simulink library "simp_vd_lib"  (R2022b)
settings: Solver=VariableStepAuto  StartTime=0.0  StopTime=10.0  RelTol=1e-3
libraries: simulink x1
settings Model: Creator=LinF  LastModifiedBy=LinF

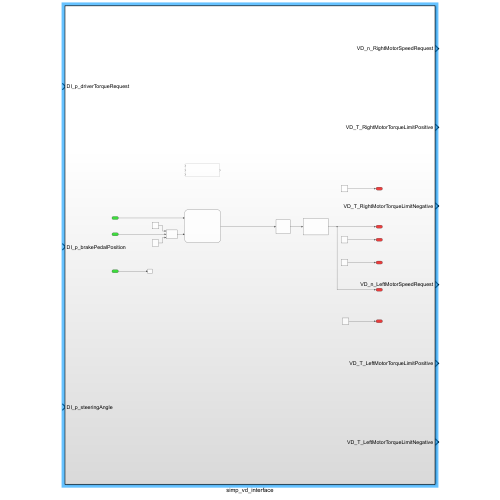
[thumbnail: Simulink's stored preview of the top-level diagram]
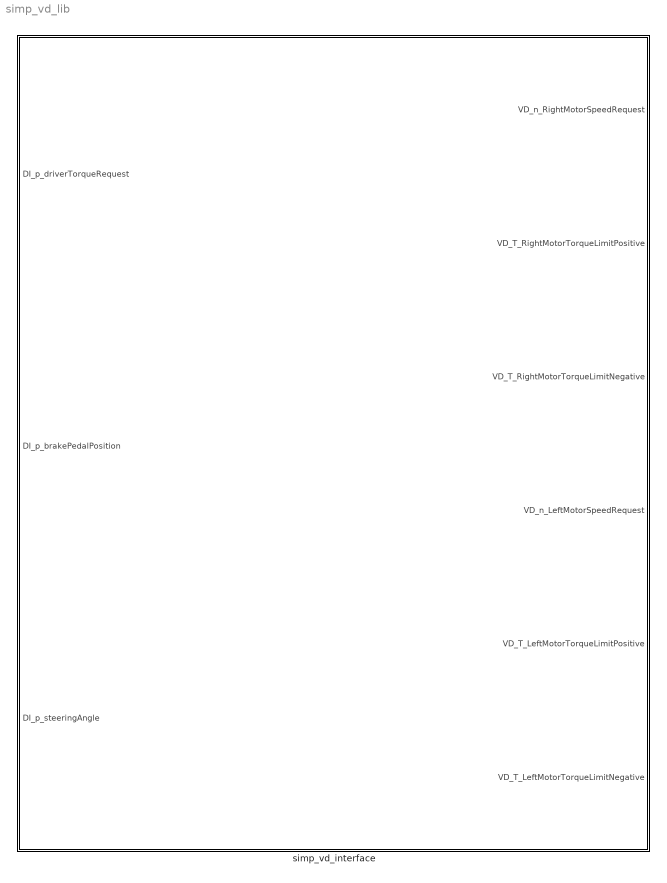
== system simp_vd_lib ==
  simp_vd_interface : Subsystem
      settings: LibrarySourceBlock=simp_vd_lib/simp_vd_interface

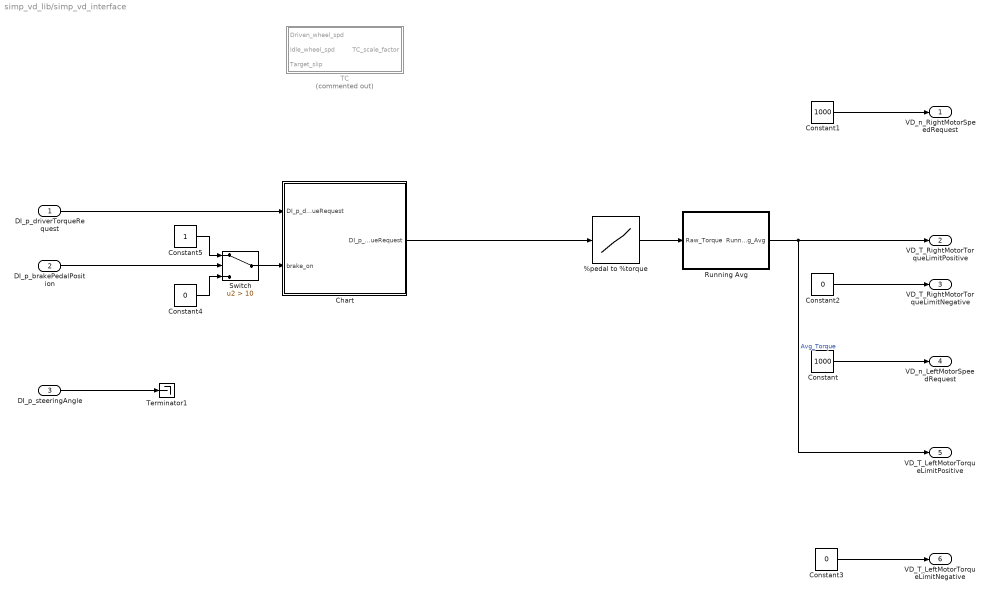
== system simp_vd_lib/simp_vd_interface ==
  DI_p_driverTorqueRequest : Inport
  DI_p_brakePedalPosition : Inport  Port=2
  DI_p_steeringAngle : Inport  Port=3
  %pedal to %torque : Lookup_n-D  NumberOfTableDimensions=1  BreakpointsForDimension1=[linspace(0,100,101)]  Table=[linspace(0,1000,101)]  InternalRulePriority=Speed  RndMeth=Simplest
  Chart : Stateflow chart  TreatAsAtomicUnit=on
  Constant : Constant  Value=1000
  Constant1 : Constant  Value=1000
  Constant2 : Constant  Value=0
  Constant3 : Constant  Value=0
  Constant4 : Constant  Value=0
  Constant5 : Constant
  Running Avg : Subsystem
  Switch : Switch  Criteria=u2 > Threshold  Threshold=10  SaturateOnIntegerOverflow=off  InputSameDT=off
  TC : Subsystem  Commented=on
  Terminator1 : Terminator
  VD_n_RightMotorSpeedRequest : Outport
  VD_T_RightMotorTorqueLimitPositive : Outport  Port=2
  VD_T_RightMotorTorqueLimitNegative : Outport  Port=3
  VD_n_LeftMotorSpeedRequest : Outport  Port=4
  VD_T_LeftMotorTorqueLimitPositive : Outport  Port=5
  VD_T_LeftMotorTorqueLimitNegative : Outport  Port=6
  wires:
  Chart/1(DI_p_motorTorqueRequest) -> %pedal to %torque/1
  Running Avg/1(Running_Avg) -> VD_T_RightMotorTorqueLimitPositive/1, VD_T_LeftMotorTorqueLimitPositive/1  "Avg_Torque"
  %pedal to %torque/1 -> Running Avg/1(Raw_Torque)
  DI_p_driverTorqueRequest/1 -> Chart/1(DI_p_driverTorqueRequest)
  DI_p_brakePedalPosition/1 -> Switch/2
  Switch/1 -> Chart/2(brake_on)
  Constant5/1 -> Switch/1
  Constant4/1 -> Switch/3
  Constant3/1 -> VD_T_LeftMotorTorqueLimitNegative/1
  Constant2/1 -> VD_T_RightMotorTorqueLimitNegative/1
  Constant1/1 -> VD_n_RightMotorSpeedRequest/1
  Constant/1 -> VD_n_LeftMotorSpeedRequest/1
  DI_p_steeringAngle/1 -> Terminator1/1

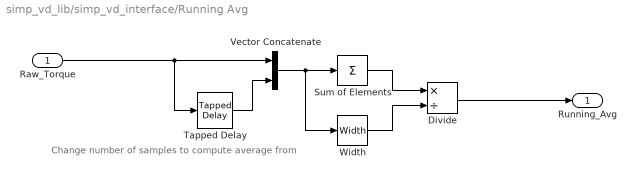
== system simp_vd_lib/simp_vd_interface/Running Avg ==
  note: Change number of samples to compute average from
  Raw_Torque : Inport
  Divide : Product  Inputs=*/
  Sum of Elements : Sum  Inputs=+
  Tapped Delay : simulink/Discrete/Tapped Delay  vinit=0  samptime=-1  NumDelays=10  DelayOrder=Oldest  includeCurrent=off
  Vector Concatenate : Concatenate
  Width : Width
  Running_Avg : Outport
  wires:
  Sum of Elements/1 -> Divide/1
  Tapped Delay/1 -> Vector Concatenate/2
  Width/1 -> Divide/2
  Raw_Torque/1 -> Tapped Delay/1, Vector Concatenate/1
  Vector Concatenate/1 -> Sum of Elements/1, Width/1
  Divide/1 -> Running_Avg/1

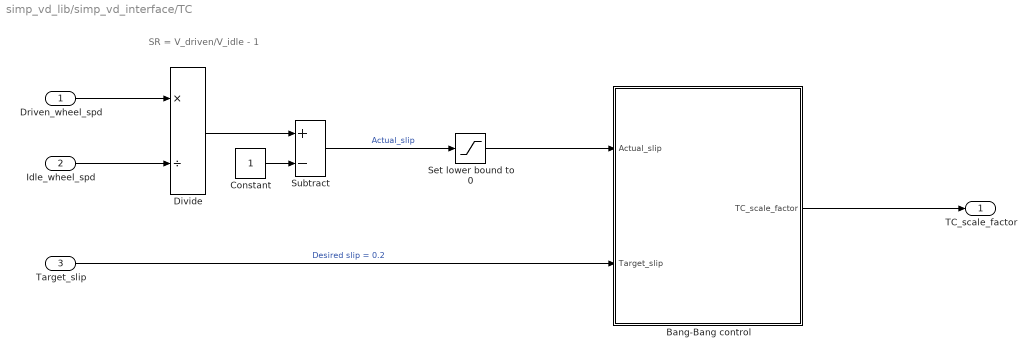
== system simp_vd_lib/simp_vd_interface/TC ==
  note: SR = V_driven/V_idle - 1
  Driven_wheel_spd : Inport
  Idle_wheel_spd : Inport  Port=2
  Target_slip : Inport  Port=3
  Bang-Bang control : Stateflow chart  TreatAsAtomicUnit=on
  Constant : Constant
  Divide : Product  Inputs=*/
  Set lower bound to 0 : Saturate  UpperLimit=inf  LowerLimit=0
  Subtract : Sum  Inputs=+-
  TC_scale_factor : Outport
  wires:
  Bang-Bang control/1(TC_scale_factor) -> TC_scale_factor/1
  Subtract/1 -> Set lower bound to 0/1  "Actual_slip"
  Target_slip/1 -> Bang-Bang control/2(Target_slip)  "Desired slip = 0.2"
  Idle_wheel_spd/1 -> Divide/2
  Driven_wheel_spd/1 -> Divide/1
  Divide/1 -> Subtract/1
  Constant/1 -> Subtract/2
  Set lower bound to 0/1 -> Bang-Bang control/1(Actual_slip)

== stateflow chart simp_vd_lib/simp_vd_interface/TC/Bang-Bang control ==
  state TC_off
    en, du:
    TC_scale_factor = 1;
  state TC_on
    en, du:
    TC_scale_factor = 0;
  (default) -> TC_off
  TC_off -> TC_on : [after(50,msec) && Actual_slip > Target_slip]
  TC_on -> TC_off : [after(50,msec) && Actual_slip <= Target_slip]
  data: Actual_slip input; Target_slip input; TC_scale_factor output

== stateflow chart simp_vd_lib/simp_vd_interface/Chart ==
  state Run
    en, du:
    DI_p_motorTorqueRequest = DI_p_driverTorqueRequest;
  state Stop
    en, du:
    DI_p_motorTorqueRequest = 0;
  (default) -> Run
  Run -> Stop : [DI_p_driverTorqueRequest >= 20 && brake_on]
  Stop -> Run : [DI_p_driverTorqueRequest < 5 && ~brake_on]
  data: DI_p_driverTorqueRequest input; brake_on input; DI_p_motorTorqueRequest output
